simulink model "Gyroscope"  (R2024b)
settings: Solver=VariableStepAuto  StartTime=0.0  StopTime=10000.0  RelTol=1e-3
undefined symbols (not defined in the file or in its folder): flag, sens
settings Model: Creator=filippocamaleonte  LastModifiedBy=filippocamaleonte

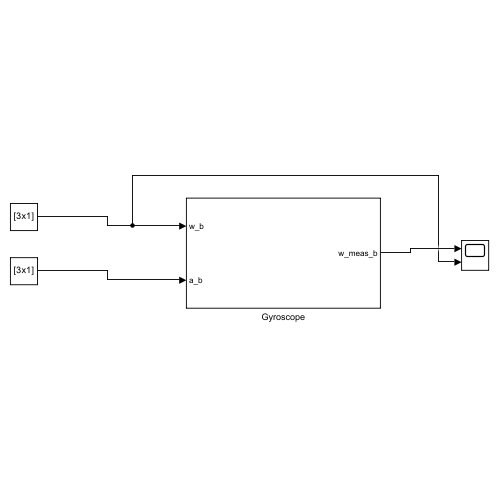
[thumbnail: Simulink's stored preview of the top-level diagram]
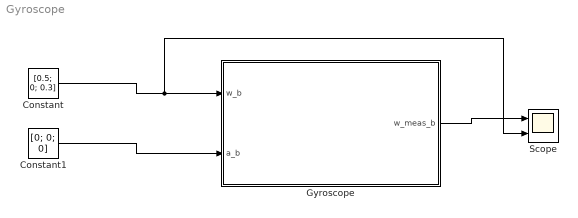
== system Gyroscope ==
  Constant : Constant  Value=[0.5; 0; 0.3]
  Constant1 : Constant  Value=[0; 0; 0]
  Gyroscope : Subsystem
  Scope : Scope  NumInputPorts=2
  wires:
  Constant/1 -> Scope/2, Gyroscope/1(w_b)
  Constant1/1 -> Gyroscope/2(a_b)
  Gyroscope/1(w_meas_b) -> Scope/1

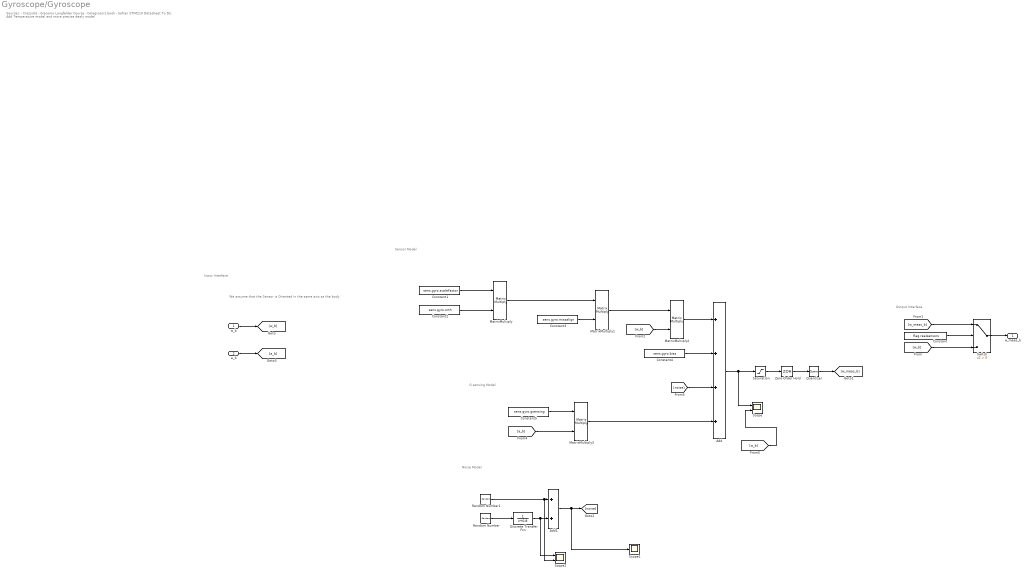
== system Gyroscope/Gyroscope ==
  note: Sensor Model
  note: Noise Model
  note: Input Interface
  note: G sensing Model
  note: Sources:
      | - Crassidis
      | - Giacomo Langfelder Course
      | - Colagrossi's book
      | - Safran STIM210 Datasheet
      |
      | To Do:
      | Add Temperature model and more precise dealy model
  note: We assume that the Sensor is Oriented in the same axis as the body
  note: Output Interface
  w_b : Inport
  a_b : Inport  Port=2
  Add : Sum  Inputs=++++
  Add1 : Sum
  Constant : Constant  Value=flag.realsensors
  Constant1 : Constant  Value=sens.gyro.scaleFactor
  Constant2 : Constant  Value=sens.gyro.orth
  Constant3 : Constant  Value=sens.gyro.missalign
  Constant4 : Constant  Value=sens.gyro.bias
  Constant5 : Constant  Value=sens.gyro.gsensing
  Discrete Transfer Fcn : DiscreteTransferFcn  Numerator=1  Denominator=[1 0.8]
  MatrixMultiply{,1..3} (4 alike) : Product  Multiplication=Matrix(*)
  Quantizer : Quantizer  QuantizationInterval=sens.gyro.ADC.quanta
  Random Number : RandomNumber  Variance=sens.gyro.biasInstability  SampleTime=1/sens.gyro.freq
  Random Number1 : RandomNumber  Variance=sens.gyro.arw  SampleTime=1/sens.gyro.freq
  Saturation : Saturate  UpperLimit=sens.gyro.saturation  LowerLimit=-sens.gyro.saturation
  Scope : Scope  NumInputPorts=2
  Scope1 : Scope
  Scope2 : Scope  NumInputPorts=2
  Switch : Switch  Criteria=u2 > Threshold  SaturateOnIntegerOverflow=off  InputSameDT=off
  Zero-Order Hold : ZeroOrderHold  SampleTime=1/sens.gyro.freq
  w_meas_b : Outport
  wires:
  Switch/1 -> w_meas_b/1
  Constant/1 -> Switch/2
  [w_meas_b] -> Switch/1
  [w_b] -> Switch/3
  w_b/1 -> [w_b]
  Quantizer/1 -> [w_meas_b]
  Zero-Order Hold/1 -> Quantizer/1
  Saturation/1 -> Zero-Order Hold/1
  MatrixMultiply/1 -> MatrixMultiply1/1
  MatrixMultiply1/1 -> MatrixMultiply2/1
  Constant1/1 -> MatrixMultiply/1
  Constant2/1 -> MatrixMultiply/2
  Constant3/1 -> MatrixMultiply1/2
  [w_b] -> MatrixMultiply2/2
  MatrixMultiply2/1 -> Add/1
  Add/1 -> Scope/1, Saturation/1
  Constant4/1 -> Add/2
  Add1/1 -> Scope1/1, [noise]
  [noise] -> Add/3
  MatrixMultiply3/1 -> Add/4
  a_b/1 -> [a_b]
  [a_b] -> MatrixMultiply3/2
  Constant5/1 -> MatrixMultiply3/1
  Discrete Transfer Fcn/1 -> Scope2/1, Add1/2
  Random Number/1 -> Discrete Transfer Fcn/1
  Random Number1/1 -> Scope2/2, Add1/1
  [w_b] -> Scope/2
